simulink model "Pacejka_longitudinal_tyre_model"  (R2024b)
settings: Solver=FixedStepAuto  StartTime=0.0  StopTime=10.0  FixedStep=0.01  RelTol=1e-3
values from neighbouring files (symbols this model uses):
  a1 = -1e-5    (= -1e-05)    [Pacejka_lateral_parameters.m]
  a2 = 1.25    [Pacejka_lateral_parameters.m]
  B = 0.1453    [Pacejka_lateral_parameters.m]
  C = 1.5511    [Pacejka_lateral_parameters.m]
settings Model: Creator=jayku  LastModifiedBy=jayku

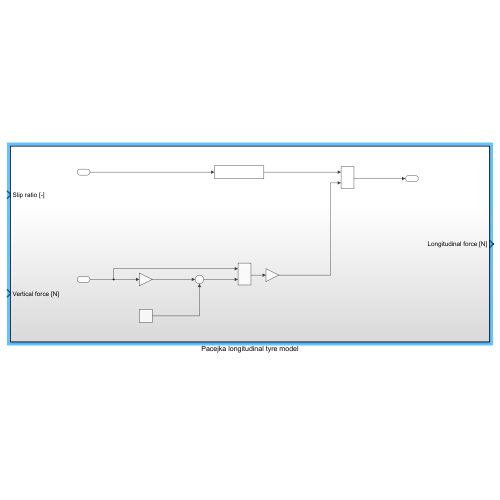
[thumbnail: Simulink's stored preview of the top-level diagram]
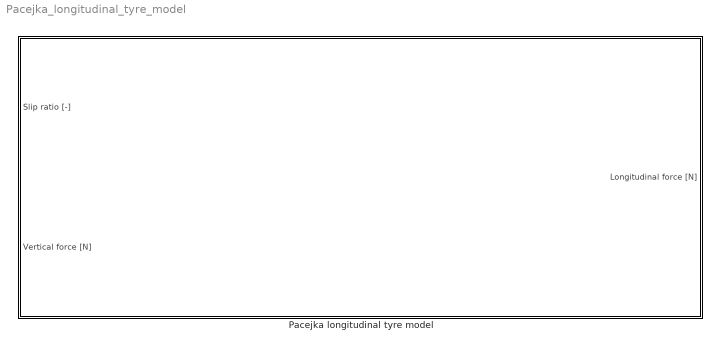
== system Pacejka_longitudinal_tyre_model ==
  Pacejka longitudinal tyre model : Subsystem

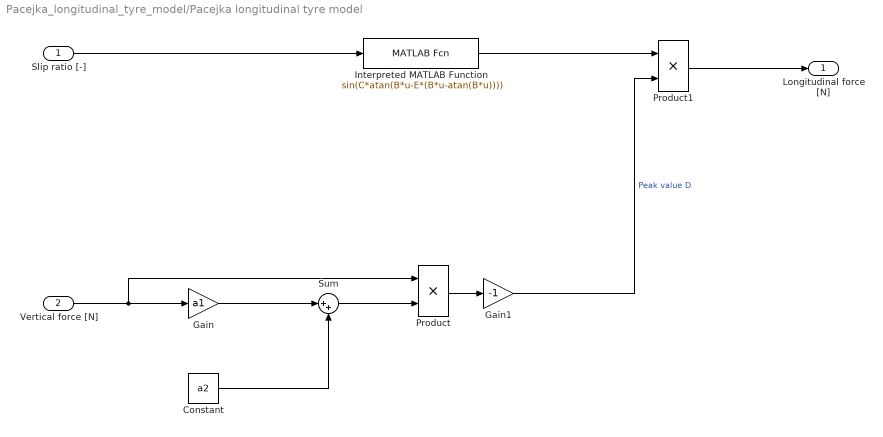
== system Pacejka_longitudinal_tyre_model/Pacejka longitudinal tyre model ==
  Slip ratio [-] : Inport
  Vertical force [N] : Inport  Port=2
  Constant : Constant  Value=a2
  Gain : Gain  Gain=a1
  Gain1 : Gain  Gain=-1
  Interpreted MATLAB Function : MATLABFcn  MATLABFcn=sin(C*atan(B*u-E*(B*u-atan(B*u))))
  Product : Product
  Product1 : Product
  Sum : Sum  Inputs=|++
  Longitudinal force [N] : Outport
  wires:
  Slip ratio [-]/1 -> Interpreted MATLAB Function/1
  Vertical force [N]/1 -> Product/1, Gain/1
  Gain/1 -> Sum/1
  Constant/1 -> Sum/2
  Sum/1 -> Product/2
  Product/1 -> Gain1/1
  Gain1/1 -> Product1/2  "Peak value D"
  Interpreted MATLAB Function/1 -> Product1/1
  Product1/1 -> Longitudinal force [N]/1
